simulink model "Simple_Model_Packaging_2_1"  (R2022b)
settings: Solver=VariableStepAuto  StartTime=0.0  StopTime=0.01  RelTol=1e-3
InitFcn:
  | Parameter_Initialize_2
undefined symbols (not defined in the file or in its folder): gcbh, magnitude, model, rcfiltgaincompat, rsgenpoly
libraries: commdigbbndpm3 x3, commdigbbndam3 x2, commfilt2 x2, commblkintrlv2 x1, commofdm x1, commmimo x1, commblkcod2 x1, commrandsrc3 x1, simulink x1, commdigbbndfm2 x1, commseqgen3 x1
settings Model: Creator=89778  LastModifiedBy=89778

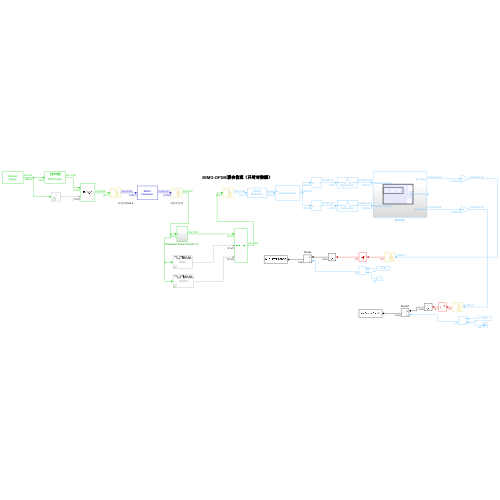
[thumbnail: Simulink's stored preview of the top-level diagram]
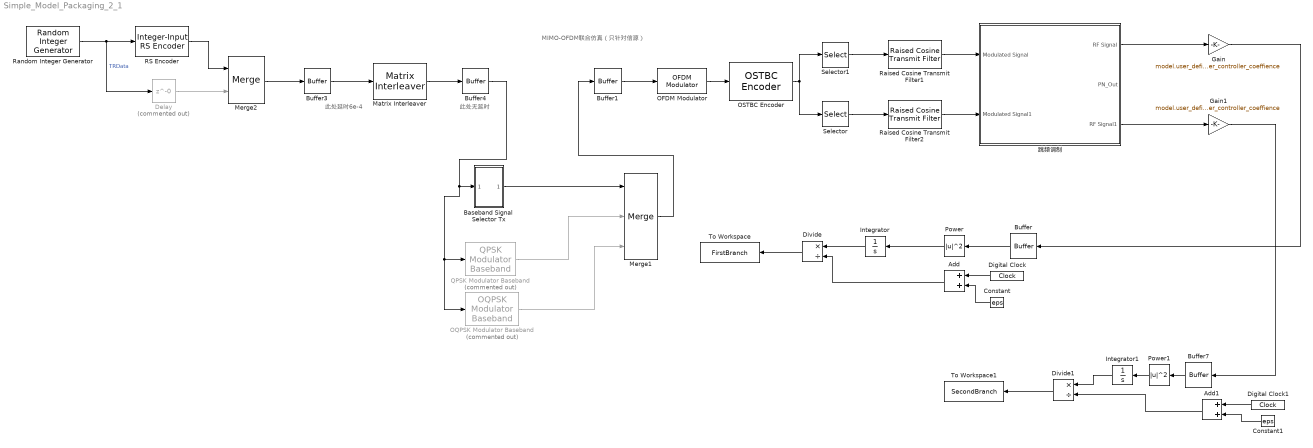
== system Simple_Model_Packaging_2_1 ==
  note: MIMO-OFDM联合仿真（只针对信源）
  note: 此处延时6e-4
  note: 此处无延时
  Add : Sum
  Add1 : Sum
  Baseband Signal Selector Tx : Subsystem
  Buffer : Buffer  N=model.parameter.Buffer.Output_buffer_size  OutputFrames=off
  Buffer1 : Buffer  N=model.parameter.Buffer1.Output_size  OutputFrames=off
  Buffer3 : Buffer  N=model.parameter.Buffer3.Output_size  OutputFrames=off
  Buffer4 : Buffer  N=model.parameter.Buffer4.Output_size  OutputFrames=off
  Buffer7 : Buffer  N=1  OutputFrames=off
  Constant : Constant  Value=eps  SampleTime=model.parameter.channel_estimate_fs
  Constant1 : Constant  Value=eps  SampleTime=model.parameter.channel_estimate_fs
  Delay : Delay  Commented=on  DelayLength=0  InitialCondition=0
  Digital Clock : DigitalClock  SampleTime=model.parameter.channel_estimate_fs
  Digital Clock1 : DigitalClock  SampleTime=model.parameter.channel_estimate_fs
  Divide : Product  Inputs=*/
  Divide1 : Product  Inputs=*/
  Gain : Gain  Gain=model.user_defined.TR.Sig_power_controller_coeffience
  Gain1 : Gain  Gain=model.user_defined.TR.Sig_power_controller_coeffience
  Integrator : Integrator
  Integrator1 : Integrator
  Matrix Interleaver : commblkintrlv2/Matrix Interleaver  StatePerturbationForJacobian=1.0e-05  Nrows=model.parameter.Matrix_Interleaver.row_nums  Ncols=model.parameter.Matrix_Interleaver.col_nums
  Merge1 : Merge  Inputs=3
  Merge2 : Merge
  OFDM Modulator : commofdm/OFDM Modulator  StatePerturbationForJacobian=1.0e-05  FFTLength=model.parameter.OFDM_Modulator.FFT_length  NumGuardBandCarriers=model.parameter.OFDM_Modulator.guard_bands_num  InsertDCNull=off  PilotInputPort=off  PilotCarrierIndices=[12; 26; 40; 54]  CyclicPrefixLength=model.parameter.OFDM_Modulator.Cyclic_prefix_length  Windowing=off  WindowLength=1  NumSymbols=model.parameter.OFDM_Modulator.OFDM_symbols_num  NumTransmitAntennas=model.parameter.OFDM_Modulator.transmit_antennas_num  SimulateUsing=Interpreted execution
  OQPSK Modulator Baseband : commdigbbndpm3/OQPSK Modulator Baseband  Commented=on  InType=Integer  Ph=0  Mapping=Gray  pulseShape=Half sine  num=[0.7071, 0.7071]  rolloff=0.2  filterSpan=10  sps=2  RateOptions=Enforce single-rate processing  outDtype=double
  OSTBC Encoder : commmimo/OSTBC Encoder  numTx=2  rate=3/4  overflowMode=Wrap  OvFlMode=off  OvFlModeLastStrValue=off
  Power : Math  Operator=magnitude^2
  Power1 : Math  Operator=magnitude^2
  QPSK Modulator Baseband : commdigbbndpm3/QPSK Modulator Baseband  Commented=on  InType=Integer  Enc=Gray  Ph=pi/4  outDtype=double  outWordLen=16  outUDDataType=sfix(16)  outFracLenMode=Best precision  outFracLen=15  outDataTypeStr=double  outLastDataTypeStr=double
  RS Encoder : commblkcod2/Integer-Input RS Encoder  n=model.parameter.RS_Encoder.Codeword_Length  k=model.parameter.RS_Encoder.Message_Length  specShortening=off  shortenedK=3  specGenPoly=off  genPoly=rsgenpoly(7,3)  specPrimPoly=off  prPoly=[1 0 1 1]  specPuncture=off  punctVec=[ones(2,1); zeros(2,1)]
  Raised Cosine Transmit Filter1 : commfilt2/Raised Cosine Transmit Filter  filtType=Square root  R=model.parameter.Raised_Cosine_Transmit_Filter1.Rolloff_factor  filtSpan=model.parameter.Raised_Cosine_Transmit_Filter1.Filter_span_in_symbols  N=model.parameter.Raised_Cosine_Transmit_Filter1.Output_samples_per_symbol  filterGain=rcfiltgaincompat(gcbh)  InputProcessing=Columns as channels (frame based)  RateOptions=Enforce single-rate processing  framing=Mute  checkCoeff=off  variableName=rcTxFilt1  checkGain=Normalized  sampMode=Mute  saveAsFlag=0  currentFiltSpan=10  D=(10)/2  launchFVT=on  roundingMode=Floor  overflowMode=off  coeffDataTypeStr=Inherit: Same word length as input  coeffMin=[]  coeffMax=[]  coeffLastDataTypeStr=Inherit: Same word length as input  outputDataTypeStr=Inherit: Same as accumulator  outputMin=[]  outputMax=[]  outputLastDataTypeStr=Inherit: Same as accumulator
  Raised Cosine Transmit Filter2 : commfilt2/Raised Cosine Transmit Filter  filtType=Square root  R=model.parameter.Raised_Cosine_Transmit_Filter2.Rolloff_factor  filtSpan=model.parameter.Raised_Cosine_Transmit_Filter2.Filter_span_in_symbols  N=model.parameter.Raised_Cosine_Transmit_Filter2.Output_samples_per_symbol  filterGain=rcfiltgaincompat(gcbh)  InputProcessing=Columns as channels (frame based)  RateOptions=Enforce single-rate processing  framing=Mute  checkCoeff=off  variableName=rcTxFilt2  checkGain=Normalized  sampMode=Mute  saveAsFlag=0  currentFiltSpan=10  D=(10)/2  launchFVT=on  roundingMode=Floor  overflowMode=off  coeffDataTypeStr=Inherit: Same word length as input  coeffMin=[]  coeffMax=[]  coeffLastDataTypeStr=Inherit: Same word length as input  outputDataTypeStr=Inherit: Same as accumulator  outputMin=[]  outputMax=[]  outputLastDataTypeStr=Inherit: Same as accumulator
  Random Integer Generator : commrandsrc3/Random Integer Generator  SetSize=model.parameter.Random_Integer_Generator.SetSize  SeedSource=Auto  Seed=4  SampleTime=model.parameter.Random_Integer_Generator.Random_Sample_Time  SamplesPerFrame=model.parameter.Random_Integer_Generator.Samples_per_frame  OutputDataType=double  SimulateUsing=Interpreted execution
  Selector : Selector  NumberOfDimensions=2  InputPortWidth=3  IndexOptions=Index vector (dialog),Index vector (dialog)  Indices=[1:272],2  OutputSizes=1,1
  Selector1 : Selector  NumberOfDimensions=2  InputPortWidth=3  IndexOptions=Index vector (dialog),Index vector (dialog)  Indices=[1:272],1  OutputSizes=1,1
  To Workspace : ToWorkspace  VariableName=FirstBranch  SaveFormat=Timeseries  SampleTime=-1
  To Workspace1 : ToWorkspace  VariableName=SecondBranch  SaveFormat=Timeseries  SampleTime=-1
  跳频调制 : Subsystem
  wires:
  Selector/1 -> Raised Cosine Transmit Filter2/1
  Selector1/1 -> Raised Cosine Transmit Filter1/1
  Digital Clock/1 -> Add/1
  Add/1 -> Divide/2
  Constant/1 -> Add/2
  Integrator/1 -> Divide/1
  Power/1 -> Integrator/1
  Buffer/1 -> Power/1
  Divide/1 -> To Workspace/1
  Matrix Interleaver/1 -> Buffer4/1
  Buffer1/1 -> OFDM Modulator/1
  OFDM Modulator/1 -> OSTBC Encoder/1
  OSTBC Encoder/1 -> Selector1/1, Selector/1
  Raised Cosine Transmit Filter1/1 -> 跳频调制/1(Modulated Signal)
  Raised Cosine Transmit Filter2/1 -> 跳频调制/2(Modulated Signal1)
  跳频调制/1(RF Signal) -> Gain/1
  跳频调制/3(RF Signal1) -> Gain1/1
  Add1/1 -> Divide1/2
  Digital Clock1/1 -> Add1/1
  Integrator1/1 -> Divide1/1
  Power1/1 -> Integrator1/1
  Buffer7/1 -> Power1/1
  Divide1/1 -> To Workspace1/1
  Constant1/1 -> Add1/2
  Random Integer Generator/1 -> Delay/1, RS Encoder/1  "TRData"
  OQPSK Modulator Baseband/1 -> Merge1/3
  Baseband Signal Selector Tx/1(Out1) -> Merge1/1
  QPSK Modulator Baseband/1 -> Merge1/2
  Buffer3/1 -> Matrix Interleaver/1
  Buffer4/1 -> OQPSK Modulator Baseband/1, QPSK Modulator Baseband/1, Baseband Signal Selector Tx/1(In1)
  Merge1/1 -> Buffer1/1
  Merge2/1 -> Buffer3/1
  RS Encoder/1 -> Merge2/1
  Delay/1 -> Merge2/2
  Gain/1 -> Buffer/1
  Gain1/1 -> Buffer7/1

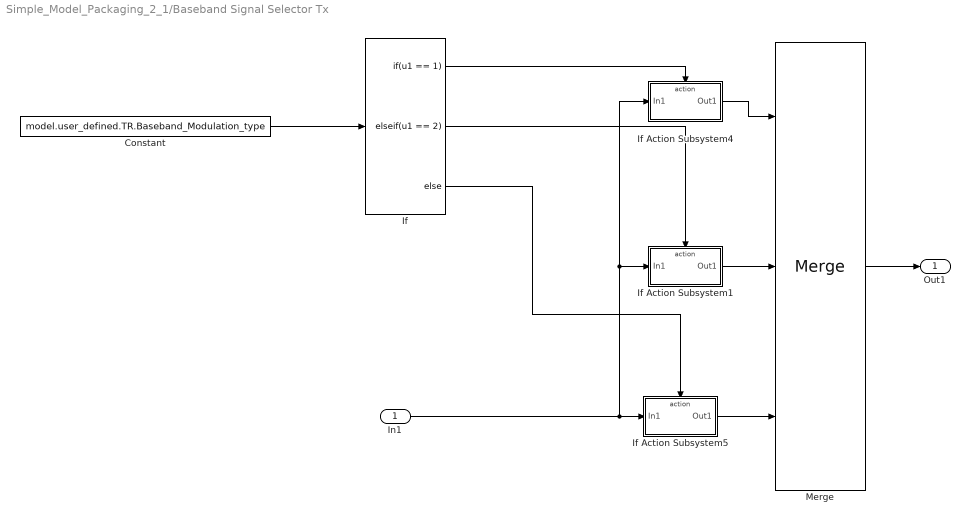
== system Simple_Model_Packaging_2_1/Baseband Signal Selector Tx ==
  In1 : Inport
  Constant : Constant  Value=model.user_defined.TR.Baseband_Modulation_type
  If : If  IfExpression=u1 == 1  ElseIfExpressions=u1 == 2
  If Action Subsystem1 : Subsystem  TreatAsAtomicUnit=on
  If Action Subsystem4 : Subsystem  TreatAsAtomicUnit=on
  If Action Subsystem5 : Subsystem  TreatAsAtomicUnit=on
  Merge : Merge  Inputs=3
  Out1 : Outport
  wires:
  If Action Subsystem5/1(Out1) -> Merge/3
  Constant/1 -> If/1
  Merge/1 -> Out1/1
  If/3 -> If Action Subsystem5/Action
  If/1 -> If Action Subsystem4/Action
  If/2 -> If Action Subsystem1/Action
  If Action Subsystem1/1(Out1) -> Merge/2
  If Action Subsystem4/1(Out1) -> Merge/1
  In1/1 -> If Action Subsystem4/1(In1), If Action Subsystem1/1(In1), If Action Subsystem5/1(In1)

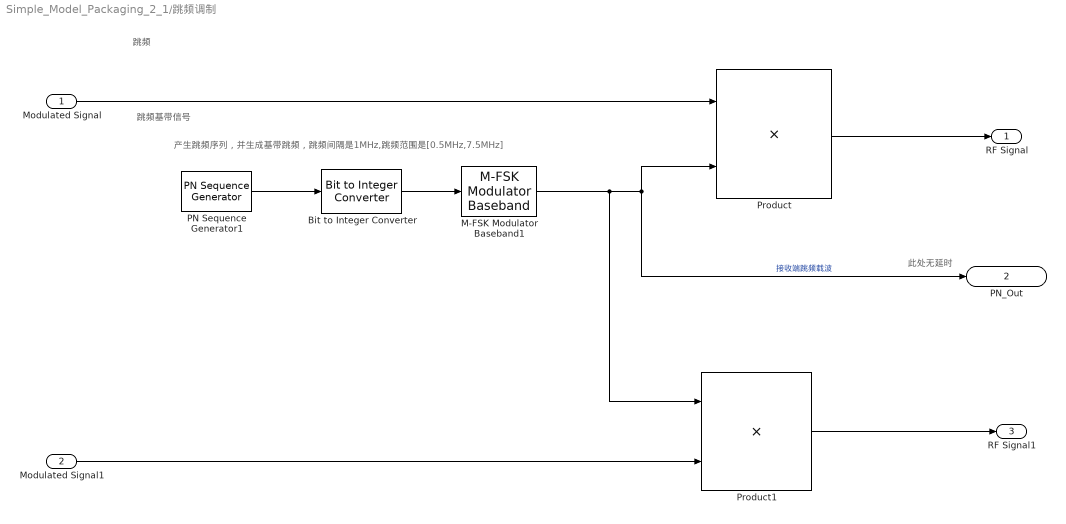
== system Simple_Model_Packaging_2_1/跳频调制 ==
  note: 跳频
  note: 此处无延时
  note: 跳频基带信号
  note: 产生跳频序列，并生成基带跳频，跳频间隔是1MHz,跳频范围是[0.5MHz,7.5MHz]
  Modulated Signal : Inport
  Modulated Signal1 : Inport  Port=2
  Bit to Integer Converter : simulink/Logic and Bit Operations/Bit to Integer Converter  nbits=model.parameter.Bit_to_Integer_Converter.M  bitOrder=MSB first  signedOutputValues=Unsigned  outDtype=double  outDtypeSigned=Inherit via internal rule
  M-FSK Modulator Baseband1 : commdigbbndfm2/M-FSK Modulator Baseband  M=model.parameter.M_FSK_Modulator_Baseband1.M_ary_number  InType=Integer  Enc=Gray  freqSep=model.parameter.M_FSK_Modulator_Baseband1.Frequency_separation  phaseType=Continuous  numSamp=model.parameter.M_FSK_Modulator_Baseband1.Samples_per_symbol  RateOptions=Enforce single-rate processing  outDataType=double
  PN Sequence Generator1 : commseqgen3/PN Sequence Generator  poly=model.parameter.PN_Sequence_Generator1.Generator_polynomial  ini_sta=model.parameter.PN_Sequence_Generator1.Initial_states  outBitMaskSource=Dialog parameter  shift=0  outVarSiz=off  maxOutSizeMode=Dialog parameter  maxOutSize=[10 1]  Ts=model.parameter.PN_Sequence_Generator1.Sample_time  sampPerFrame=model.parameter.PN_Sequence_Generator1.Samples_per_frame  reset=off  bitPackedOutputs=off  outDataType=double  numPackedBits=5  bitPackDataSigned=off  bitPackedOutDType=double
  Product : Product
  Product1 : Product
  RF Signal : Outport
  PN_Out : Outport  Port=2
  RF Signal1 : Outport  Port=3
  wires:
  M-FSK Modulator Baseband1/1 -> PN_Out/1, Product/2, Product1/1  "接收端跳频载波"
  Product/1 -> RF Signal/1
  Product1/1 -> RF Signal1/1
  Modulated Signal1/1 -> Product1/2
  Modulated Signal/1 -> Product/1
  PN Sequence Generator1/1 -> Bit to Integer Converter/1
  Bit to Integer Converter/1 -> M-FSK Modulator Baseband1/1

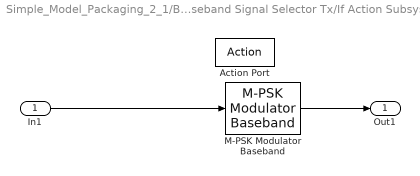
== system Simple_Model_Packaging_2_1/Baseband Signal Selector Tx/If Action Subsystem1 ==
  In1 : Inport
  Action Port : ActionPort  ActionPortLabel=elseif(u1 == 2)
  M-PSK Modulator Baseband : commdigbbndpm3/M-PSK Modulator Baseband  M=model.user_defined.Rectangular_QAM_Modulator_Baseband.M_Number  InType=Integer  Enc=Gray  Mapping=[0:7]  Ph=0  outDtype=double  outWordLen=16  outUDDataType=sfix(16)  outFracLenMode=Best precision  outFracLen=15  outDataTypeStr=double  outLastDataTypeStr=double
  Out1 : Outport
  wires:
  M-PSK Modulator Baseband/1 -> Out1/1
  In1/1 -> M-PSK Modulator Baseband/1

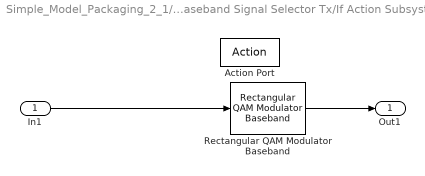
== system Simple_Model_Packaging_2_1/Baseband Signal Selector Tx/If Action Subsystem4 ==
  In1 : Inport
  Action Port : ActionPort  ActionPortLabel=if(u1 == 1)
  Rectangular QAM Modulator Baseband : commdigbbndam3/Rectangular QAM Modulator Baseband  M=model.user_defined.Rectangular_QAM_Modulator_Baseband.M_Number  InType=Integer  Enc=Gray  Mapping=[0:15]  PowType=Min. distance between symbols  MinDist=model.parameter.Rectangular_QAM_Modulator_Baseband.Minimum_distance  AvgPow=1  PeakPow=1  Ph=0  outDtype=double  outWordLen=16  outUDDataType=sfix(16)  outFracLenMode=Best precision  outFracLen=15  outDataTypeStr=double  outLastDataTypeStr=double
      settings: LibrarySourceBlock=|
      | commhdldigbbndam/Rectangular QAM
      | Modulator
      | Baseband
  Out1 : Outport
  wires:
  Rectangular QAM Modulator Baseband/1 -> Out1/1
  In1/1 -> Rectangular QAM Modulator Baseband/1

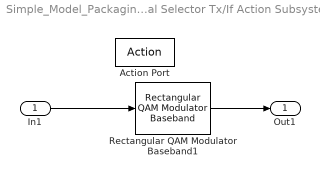
== system Simple_Model_Packaging_2_1/Baseband Signal Selector Tx/If Action Subsystem5 ==
  In1 : Inport
  Action Port : ActionPort  ActionPortLabel=else
  Rectangular QAM Modulator Baseband1 : commdigbbndam3/Rectangular QAM Modulator Baseband  M=model.user_defined.Rectangular_QAM_Modulator_Baseband.M_Number  InType=Integer  Enc=Gray  Mapping=[0:15]  PowType=Min. distance between symbols  MinDist=2  AvgPow=1  PeakPow=1  Ph=0  outDtype=double  outWordLen=16  outUDDataType=sfix(16)  outFracLenMode=Best precision  outFracLen=15  outDataTypeStr=double  outLastDataTypeStr=double
      settings: LibrarySourceBlock=|
      | commhdldigbbndam/Rectangular QAM
      | Modulator
      | Baseband
  Out1 : Outport
  wires:
  In1/1 -> Rectangular QAM Modulator Baseband1/1
  Rectangular QAM Modulator Baseband1/1 -> Out1/1
